simulink model "prb8"  (R2020a)
settings: Solver=VariableStepAuto  StartTime=0.0  StopTime=10.0  RelTol=1e-3
settings Model: Creator=Riyansh  LastModifiedBy=Riyansh

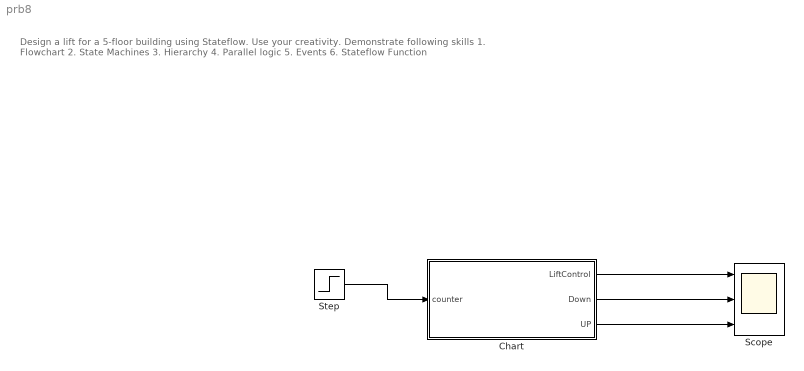
== system prb8 ==
  note: Design a lift for a 5-floor building using Stateflow. Use your creativity.
      | Demonstrate following skills
      | 1. Flowchart
      | 2. State Machines
      | 3. Hierarchy
      | 4. Parallel logic
      | 5. Events
      | 6. Stateflow Function
  Chart : Stateflow chart  TreatAsAtomicUnit=on
  Scope : Scope  NumInputPorts=3
  Step : Step  SampleTime=0
  wires:
  Chart/1(LiftControl) -> Scope/1
  Chart/3(UP) -> Scope/3
  Chart/2(Down) -> Scope/2
  Step/1 -> Chart/1(counter)

== stateflow chart prb8/Chart ==
  state LiftControl1 [parallel]
    during: LiftControl;
    settings: executionOrder=1
    state Normal
    state Upshift
      entry: count=0;
      during: count=count+1;
    state Downshift
      entry: count=0;
      during: count=count-1;
    (default) -> Normal : {count=0}
    Normal -> Downshift [order 1] : [count>5]
    Normal -> Upshift [order 2] : [count<5]
    Downshift -> Normal : [count<5]
    Upshift -> Normal : [count>5]
  state LiftControl [parallel]
    settings: executionOrder=2
    state Floor_1
      entry: counter=1;
    state Floor_2
      entry:counter=2;
    state Floor_3
      entry:counter=3;
    state Floor_4
      entry:counter=4;
    state Floor_5
      entry:counter=5;
    (default) -> Floor_1
    Floor_3 -> Floor_4 [order 2] : [UP]
    Floor_4 -> Floor_5 [order 1]
    Floor_2 -> Floor_3 [order 1] : [UP]
    Floor_1 -> Floor_2 : [UP]
    Floor_2 -> Floor_1 [order 2] : [Down]
    Floor_4 -> Floor_3 [order 2] : [Down]
    Floor_5 -> Floor_4
    Floor_3 -> Floor_2 [order 1] : [Down]
  (default) -> LiftControl1
  data: count local; counter input; LiftControl output; Down output; UP output
